simulink model "sim_transmission"  (R2018a)
settings: Solver=VariableStepAuto  StartTime=0.0  StopTime=10.0  RelTol=1e-3
libraries: dspvision x2, commchan3 x1
settings Model: Creator=prana  LastModifiedBy=prana

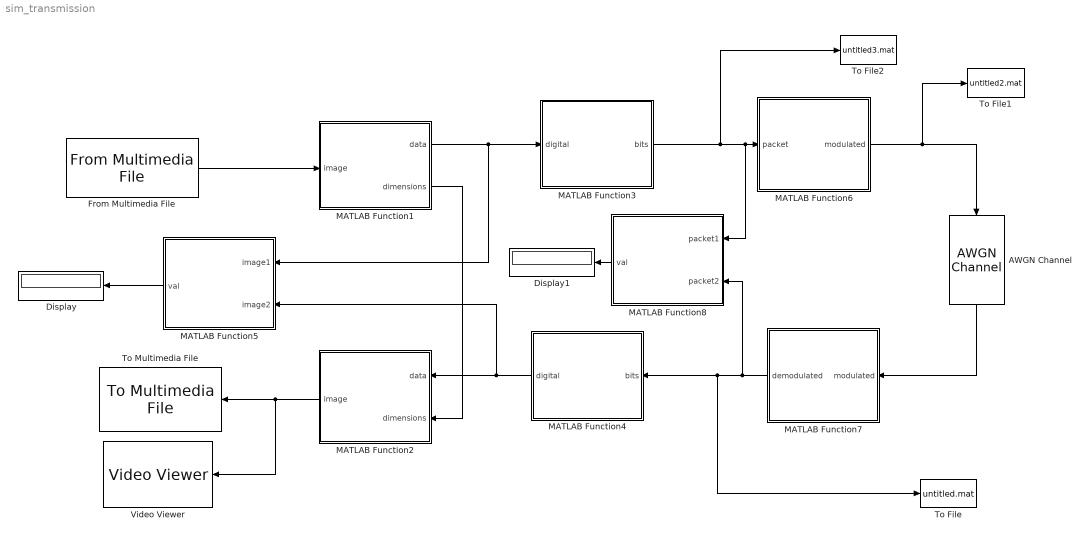
== system sim_transmission ==
  AWGN Channel : commchan3/AWGN Channel  InputProcessing=Columns as channels (frame based)  seed=67  noiseMode="Signal to noise ratio  (Eb/No)"  EbNodB=10  EsNodB=10  SNRdB=10  bitsPerSym=1  Ps=1  Tsym=1  variance=1
  Display : Display
  Display1 : Display
  From Multimedia File : dspvision/From Multimedia File  inputFilename=C:\Users\prana\Videos\2022-01-30 03-29-43.mp4  loop=on  numPlays=inf  outputStreams=Video only  videoDataType=uint8  audioDataType=int16  inheritSampleTime=on  userDefinedSampleTime=1/30  noAudioOutput=off  isIntensityVideo=off  fourcc=RGB  colorVideoFormat=One multidimensional signal  outputEOF=off  dataOrg=Column-major  audioFrameSize=1024  computeAudioFrameSize=off  outSamplingMode=Sample based
      settings: SourceProductBaseCode=VP
  MATLAB Function1 : MATLAB Function  TreatAsAtomicUnit=on
  MATLAB Function2 : MATLAB Function  TreatAsAtomicUnit=on
  MATLAB Function3 : MATLAB Function  TreatAsAtomicUnit=on
  MATLAB Function4 : MATLAB Function  TreatAsAtomicUnit=on
  MATLAB Function5 : MATLAB Function  TreatAsAtomicUnit=on
  MATLAB Function6 : MATLAB Function  TreatAsAtomicUnit=on
  MATLAB Function7 : MATLAB Function  TreatAsAtomicUnit=on
  MATLAB Function8 : MATLAB Function  TreatAsAtomicUnit=on
  To File : ToFile  MatrixName=demodulated  SaveFormat=Timeseries
  To File1 : ToFile  Filename=untitled2.mat  MatrixName=modulated  SaveFormat=Timeseries
  To File2 : ToFile  Filename=untitled3.mat  MatrixName=image  SaveFormat=Timeseries
  To Multimedia File : dspvision/To Multimedia File  outputFilename=C:\Users\prana\OneDrive\Documents\GitHub\Telecommunication-Network\output.avi  streamSelection=Video only  videoCompressor=None (uncompressed)  audioCompressor=None (uncompressed)  imagePorts=One multidimensional signal  fileType=AVI  audioDatatype=Determine from input data type  fourcc=RGB  videoQuality=75  mj2000CompFactor=10
      settings: SourceProductName=Computer Vision System Toolbox  SourceProductBaseCode=VP
  Video Viewer : VideoViewer  FigPos=[644.2 595.6 417.6 304]
  wires:
  MATLAB Function2/1(image) -> To Multimedia File/1, Video Viewer/1
  MATLAB Function1/2(dimensions) -> MATLAB Function2/2(dimensions)
  MATLAB Function1/1(data) -> MATLAB Function5/1(image1), MATLAB Function3/1(digital)
  MATLAB Function4/1(digital) -> MATLAB Function5/2(image2), MATLAB Function2/1(data)
  MATLAB Function5/1(val) -> Display/1
  MATLAB Function3/1(bits) -> To File2/1, MATLAB Function8/1(packet1), MATLAB Function6/1(packet)
  MATLAB Function8/1(val) -> Display1/1
  MATLAB Function6/1(modulated) -> To File1/1, AWGN Channel/1
  AWGN Channel/1 -> MATLAB Function7/1(modulated)
  From Multimedia File/1 -> MATLAB Function1/1(image)
  MATLAB Function7/1(demodulated) -> MATLAB Function8/2(packet2), To File/1, MATLAB Function4/1(bits)

== matlab function sim_transmission/MATLAB Function1 ==
  data: image input; data output; dimensions output
function [data,dimensions]= serialize(image)
image = imresize(image,[128 128]);
dimensions=size(image);
data=image(:);
end

== matlab function sim_transmission/MATLAB Function2 ==
  data: data input; image output; dimensions input
function image = deserialize(data,dimensions)
    image=reshape(data,128,128,3);
end

== matlab function sim_transmission/MATLAB Function3 ==
  data: digital input; bits output
function bits=quantize_image(digital)
    size(digital)
    b = de2bi(digital,'left-msb',8)';%converting to binary(column vector) where eight bits mean a number
    %size(b)
    bits=b(:)';
end

== matlab function sim_transmission/MATLAB Function4 ==
  data: bits input; digital output
function digital=dequantize_image(bits)
    bits=reshape(bits,8,[])';
    digital = bi2de(bits,'left-msb')';%converting to binary(column vector) where eight bits mean a number
    size(digital)
end

== matlab function sim_transmission/MATLAB Function5 ==
  data: image1 input; val output; image2 input
function val=error_samples(image1,image2)
image1(1:10);
image2(1:10);
[w h c]=size(image1);
val=sum(image1(:)~=image2(:))/(w*h*c)*100;
end

== matlab function sim_transmission/MATLAB Function6 ==
  data: packet input; modulated output
%function modulated  = modulate(packet, ta, ns, fc)
function modulated  = modulate(packet)
packet=double(packet);
ta=0.2e-3;
fc=20e3;
ns=20;
% MODULATE Brief summary of this function.
% 
% Detailed explanation of this function.
% modulate packet
% ta = bit pulse duration
% ns = no of samples in one pulse
% fc = carrier freq
% use any modulation.
% but take care of BER and latency.
%Let's implement it
m = packet;
m = 2*m - 1;
% you can manually loop and assign the values to me and mo but this is fast
me = m(2:2:end);
mo = m(1:2:end);
% The rest code is same as QAM just the duration is halfed. only t changes
dt = ta/ns;
% time values note that instead of size of m, we have size of me which is half
t = dt:dt:ta*size(me, 2);
% lets make physical versions of m1 and m2
s1 = me(ceil(t/ta));
s2 = mo(ceil(t/ta));
%plot(t, s1);
%plot(t, s2);
% cosine part:
cosine = s1 .* cos(2*pi*fc*t);
% sine part:
sine = s2 .* sin(2*pi*fc*t);
modulated = cosine + sine;
% add noise say, with snr 18 dB
%modulated = awgn(modulated, 18);
%plot(t,modulated);
end

== matlab function sim_transmission/MATLAB Function7 ==
  data: modulated input; demodulated output
%function demodulated  = demodulate(modulated, ta, ns, fc)
function demodulated  = demodulate(modulated)
ta=0.2e-3;
fc=20e3;
ns=20;
% DEMODULATE Brief summary of this function.
% 
% Detailed explanation of this function.
% demodulate packet
% ta = bit pulse duration
% ns = no of samples in one pulse
% fc = carrier freq
dt=ta/ns;
t = dt:dt:dt*size(modulated,2);
% multiplying modulated signal by cos(2*pi*fc*t)
sig1 = modulated .* cos(2*pi*fc*t);
% multiplying modulated signal by sin(2*pi*fc*t)
sig2 = modulated .* sin(2*pi*fc*t);
% now we will apply the filter (conv):
sig1 = conv(sig1, ones(1, ns)*dt, 'same');
sig2 = conv(sig2, ones(1, ns)*dt, 'same');
% threshold as before
sig1 = sig1 > 0;
sig2 = sig2 > 0;
%plot(t, sig1);
%plot(t, sig2);
% sample
sampling_times = ta/2:ta:dt*size(modulated, 2);
m1_reconstructed = sig1(floor(sampling_times/dt));
m1_reconstructed = m1_reconstructed > 0;
m2_reconstructed = sig2(floor(sampling_times/dt));
m2_reconstructed = m2_reconstructed > 0;
% combining them,
% odd places
m_reconstructed = [ m2_reconstructed ; m1_reconstructed]; 
% even places
m_final = m_reconstructed(:)';
demodulated=uint8(m_final);
end

== matlab function sim_transmission/MATLAB Function8 ==
  data: packet1 input; val output; packet2 input
function val=error_samples(packet1,packet2)
[w h c]=size(packet1);
%val=sum(packet1(:)~=packet2(:))/(w*h*c)*100;
val=sum(packet1(:)~=packet2(:));
all(packet1(:)==packet2(:))
end
